simulink model "DGL2slx"  (R2015b)
settings: Solver=ode3  StartTime=0.0  StopTime=10.0  FixedStep=0.001  RelTol=1e-3
settings Model: Creator=Andreas  LastModifiedBy=Wolfgang
settings DataIOCC: SaveFormat=Array
settings DebuggingCC: SolverPrmCheckMsg=warning
settings HardwareCC: ProdBitPerPointer=32  ProdLargestAtomicFloat=None  ProdIntDivRoundTo=Undefined  ProdEndianess=Unspecified  ProdWordSize=32  ProdHWDeviceType=32-bit Generic
settings GRTTargetCC: GeneratePreprocessorConditionals=Disable all
settings ConfigComp: CovModelRefEnable=Off  CovSFcnEnable=off

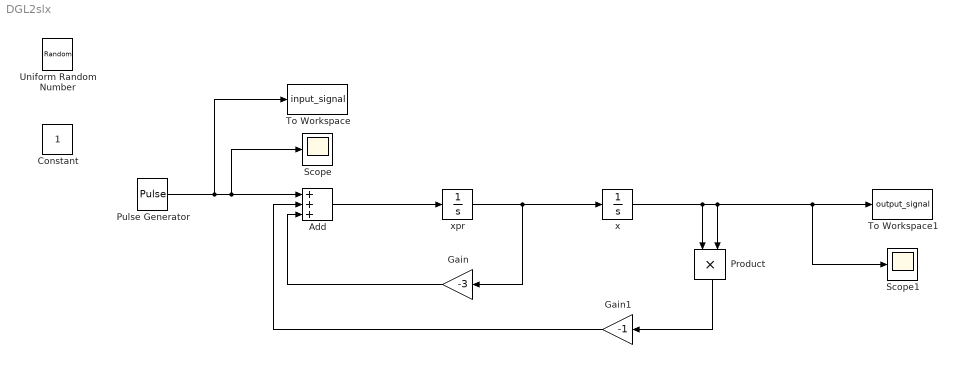
== system DGL2slx ==
  Add : Sum  Inputs=+++
  Constant : Constant
  Gain : Gain  Gain=-3
  Gain1 : Gain  Gain=-1
  Product : Product
  Pulse Generator : DiscretePulseGenerator  PulseType=Time based  Period=5  PulseWidth=5
  Scope : Scope
  Scope1 : Scope
  To Workspace : ToWorkspace  VariableName=input_signal  SampleTime=-1
  To Workspace1 : ToWorkspace  VariableName=output_signal  SampleTime=-1
  Uniform Random Number : UniformRandomNumber  SampleTime=0.001
  x : Integrator
  xpr : Integrator
  wires:
  xpr/1 -> x/1, Gain/1
  x/1 -> To Workspace1/1, Scope1/1, Product/2, Product/1
  Add/1 -> xpr/1
  Pulse Generator/1 -> To Workspace/1, Scope/1, Add/1
  Gain/1 -> Add/3
  Gain1/1 -> Add/2
  Product/1 -> Gain1/1
